simulink model "gm_hdl_model_fixed_vnl"  (R2024a)
settings: Solver=FixedStepDiscrete  StartTime=0.0  StopTime=SIM_TIME  RelTol=1e-3
undefined symbols (not defined in the file or in its folder): a, b, BUFFER_LEN, c, SAMPLING_FREQ, signal_1
libraries: hdlsllib x41, simulink x16, dspsigops x15, simulink_extras x5, dsphdlxfrm2 x2, dspsrcs4 x1
(part 2 of 3)

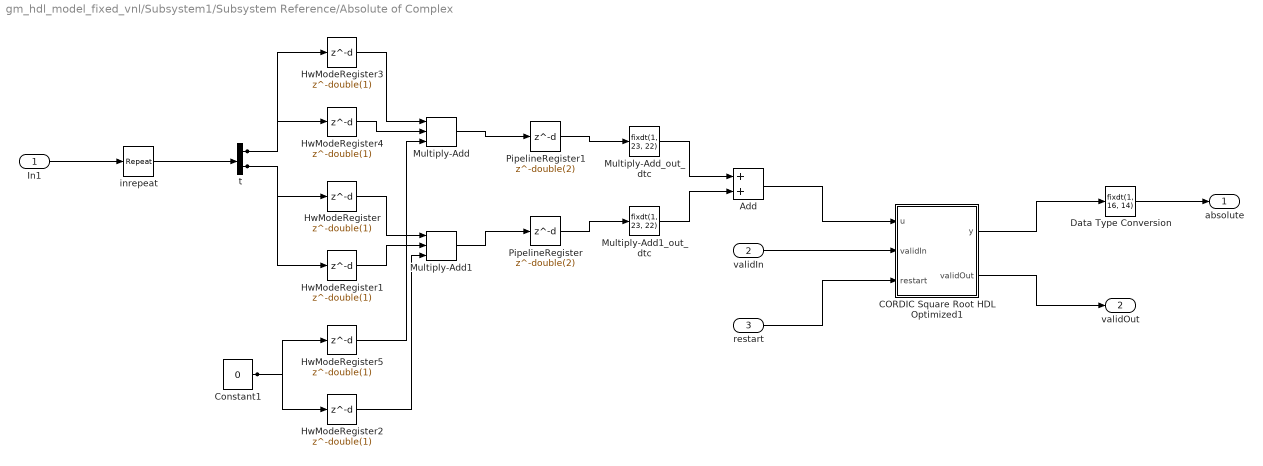
== system gm_hdl_model_fixed_vnl/Subsystem1/Subsystem Reference/Absolute of Complex ==
  In1 : Inport  OutDataTypeStr=fixdt(1, 12, 11)  PortDimensions=[2]  SampleTime=1e-08
  validIn : Inport  Port=2  OutDataTypeStr=boolean  PortDimensions=1  SampleTime=1e-08
  restart : Inport  Port=3  OutDataTypeStr=boolean  PortDimensions=1  SampleTime=1e-08
  Add : Sum  OutDataTypeStr=fixdt(1, 24, 22)  AccumDataTypeStr=fixdt(1, 24, 22)  SampleTime=5e-09
  CORDIC Square Root HDL Optimized1 : Subsystem  mask(CORDIC Square Root HDL Optimized){autoMaximumShiftVal=on, maximumShiftValue=double(10), nIterPerReg=double(1)}
      mask prompts: autoMaximumShiftVal "fixed:emblib:AutoCORDICMaxShiftValue"; maximumShiftValue "fixed:emblib:CORDICMaxShiftValue"; nIterPerReg "fixed:emblib:NumberOfIterationsPerReg"
      mask help: fixed:emblib:CORDICSquareRootHDLFullDescription
      mask Help: eval('embblk.embhelp(gcb)')
      mask Callback autoMaximumShiftVal:
      | autoMaxShiftVal = get_param(gcb,'autoMaximumShiftVal');
      | if strcmp(autoMaxShiftVal,'on')
      |     set_param(gcb,'MaskVisibilities',{'on','off','on'});
      | else
      |     set_param(gcb,'MaskVisibilities',{'on','on','on'});
      | end
      mask Display: disp('CORDIC Square Root\nHDL Optimized')
  Constant1 : Constant  Value=0  OutDataTypeStr=fixdt(1, 12, 11)  SampleTime=5e-09
  Data Type Conversion : DataTypeConversion  OutDataTypeStr=fixdt(1, 16, 14)  SampleTime=5e-09  SaturateOnIntegerOverflow=off  RndMeth=Floor
  HwModeRegister{,1..5} (6 alike) : Delay  DelayLength=double(1)  InitialCondition=0  SampleTime=5e-09
  Multiply-Add : hdlsllib/HDL Operations/Multiply-Add  Function=c+(a.*b)  datatype=fixdt(1, 25, 22)  DoSatur=off  FMA=off
  Multiply-Add1 : hdlsllib/HDL Operations/Multiply-Add  Function=c+(a.*b)  datatype=fixdt(1, 25, 22)  DoSatur=off  FMA=off
  Multiply-Add1_out_dtc : DataTypeConversion  OutDataTypeStr=fixdt(1, 23, 22)  SampleTime=5e-09  SaturateOnIntegerOverflow=off  RndMeth=Floor
  Multiply-Add_out_dtc : DataTypeConversion  OutDataTypeStr=fixdt(1, 23, 22)  SampleTime=5e-09  SaturateOnIntegerOverflow=off  RndMeth=Floor
  PipelineRegister : Delay  DelayLength=double(2)  InitialCondition=0  SampleTime=5e-09
  PipelineRegister1 : Delay  DelayLength=double(2)  InitialCondition=0  SampleTime=5e-09
  inrepeat : dspsigops/Repeat  FactorSource=Dialog parameter  N=double(2)  Nmax=16  RateOptions=Allow multirate processing  ic=0  mode=Unused parameter value
  t : Demux  Outputs=2
  absolute : Outport  SampleTime=5e-09
  validOut : Outport  Port=2  SampleTime=1e-08
  wires:
  HwModeRegister5/1 -> Multiply-Add/3
  HwModeRegister4/1 -> Multiply-Add/2
  HwModeRegister3/1 -> Multiply-Add/1
  Multiply-Add/1 -> PipelineRegister1/1
  HwModeRegister2/1 -> Multiply-Add1/3
  HwModeRegister1/1 -> Multiply-Add1/2
  HwModeRegister/1 -> Multiply-Add1/1
  Multiply-Add1/1 -> PipelineRegister/1
  PipelineRegister1/1 -> Multiply-Add_out_dtc/1
  PipelineRegister/1 -> Multiply-Add1_out_dtc/1
  t/2 -> HwModeRegister1/1, HwModeRegister/1
  t/1 -> HwModeRegister4/1, HwModeRegister3/1
  Multiply-Add_out_dtc/1 -> Add/1
  Multiply-Add1_out_dtc/1 -> Add/2
  Constant1/1 -> HwModeRegister5/1, HwModeRegister2/1
  inrepeat/1 -> t/1
  CORDIC Square Root HDL Optimized1/1(y) -> Data Type Conversion/1
  Add/1 -> CORDIC Square Root HDL Optimized1/1(u)
  Data Type Conversion/1 -> absolute/1
  CORDIC Square Root HDL Optimized1/2(validOut) -> validOut/1
  restart/1 -> CORDIC Square Root HDL Optimized1/3(restart)
  validIn/1 -> CORDIC Square Root HDL Optimized1/2(validIn)
  In1/1 -> inrepeat/1

== system gm_hdl_model_fixed_vnl/Subsystem1/Subsystem Reference/CORDIC Square Root HDL Optimized ==
  u : Inport  OutDataTypeStr=fixdt(1, 22, 20)  SampleTime=1e-08
  validIn : Inport  Port=2  OutDataTypeStr=boolean  SampleTime=1e-08
  restart : Inport  Port=3  OutDataTypeStr=boolean  SampleTime=1e-08
  Bit Shift Arithmetic : Subsystem
  Cast to Union of Types : Subsystem
  Data Type Conversion : DataTypeConversion  OutDataTypeStr=fixdt(1,22,20)
  Synchronous Subsystem : Subsystem
  y : Outport  SampleTime=1e-08
  validOut : Outport  Port=2  SampleTime=1e-08
  wires:
  Bit Shift Arithmetic/1(y) -> Data Type Conversion/1
  Cast to Union of Types/1(Cout) -> Bit Shift Arithmetic/1(u)
  Synchronous Subsystem/4(validOut) -> validOut/1
  Synchronous Subsystem/3(isZero) -> Bit Shift Arithmetic/3(isZero)
  Synchronous Subsystem/2(eOut) -> Bit Shift Arithmetic/2(e)
  Synchronous Subsystem/1(dataOut) -> Cast to Union of Types/2(Cin)
  Data Type Conversion/1 -> y/1
  restart/1 -> Synchronous Subsystem/3(restart)
  validIn/1 -> Synchronous Subsystem/2(validIn)
  u/1 -> Cast to Union of Types/1(Xref), Synchronous Subsystem/1(u)

== system gm_hdl_model_fixed_vnl/Subsystem1/Subsystem Reference/Real Divide HDL Optimized ==
  num : Inport  OutDataTypeStr=fixdt(1, 17, 14)  SampleTime=1e-08
  den : Inport  Port=2  OutDataTypeStr=fixdt(1, 17, 14)  SampleTime=5e-09
  validIn : Inport  Port=3  OutDataTypeStr=boolean  SampleTime=1e-08
  Delay1 : Delay  DelayLength=double(1)  InitialCondition=0  SampleTime=1e-08
  Delay17 : Delay  DelayLength=double(1)  InitialCondition=0  SampleTime=1e-08
  ForEach - Real Divide_instance1 : Subsystem
  Reshape to original size : Subsystem
  Verify divide sizes : Subsystem
  in1_repeat : dspsigops/Repeat  FactorSource=Dialog parameter  N=double(2)  Nmax=16  RateOptions=Allow multirate processing  ic=0  mode=Unused parameter value
  y = u(1) : Subsystem
  y : Outport  SampleTime=1e-08
  validOut : Outport  Port=2  SampleTime=1e-08
  wires:
  in1_repeat/1 -> Verify divide sizes/2(numerator)
  Verify divide sizes/2(num) -> ForEach - Real Divide_instance1/2(num)
  Verify divide sizes/1(den) -> ForEach - Real Divide_instance1/1(den)
  den/1 -> Verify divide sizes/1(denominator)
  Reshape to original size/1(z) -> Delay17/1
  y = u(1)/1(y) -> Delay1/1
  Delay17/1 -> y/1
  Delay1/1 -> validOut/1
  ForEach - Real Divide_instance1/2(validOut) -> y = u(1)/1(u)
  ForEach - Real Divide_instance1/1(y) -> Reshape to original size/1(y)
  validIn/1 -> ForEach - Real Divide_instance1/3(validIn)
  num/1 -> in1_repeat/1, Reshape to original size/2(u)

== system gm_hdl_model_fixed_vnl/Subsystem1/Subsystem Reference/Sample and Hold ==
  In : Inport  OutDataTypeStr=fixdt(1, 16, 14)
  Trigger : TriggerPort  VariantControl=(inherit)  OutDataTypeStr=boolean
  " " : Outport  InitialOutput=0
  wires:
  In/1 -> " "/1

== system gm_hdl_model_fixed_vnl/Subsystem1/Subsystem Reference/Sample and Hold1 ==
  In : Inport  OutDataTypeStr=fixdt(1, 18, 10)
  Trigger : TriggerPort  VariantControl=(inherit)  OutDataTypeStr=boolean
  " " : Outport  InitialOutput=0
  wires:
  In/1 -> " "/1

== system gm_hdl_model_fixed_vnl/Subsystem1/Subsystem Reference/Sample and Hold2 ==
  In : Inport  OutDataTypeStr=fixdt(1, 22, 20)
  Trigger : TriggerPort  VariantControl=(inherit)  OutDataTypeStr=boolean
  " " : Outport  InitialOutput=0
  wires:
  In/1 -> " "/1

== system gm_hdl_model_fixed_vnl/Subsystem1/Subsystem Reference/Select_Freq ==
  enb : Inport  OutDataTypeStr=boolean  PortDimensions=1  SampleTime=1e-08
  AND : Logic  AllPortsSameDT=off  OutDataTypeStr=boolean  SampleTime=1e-08
  Constant : Constant  Value=0  OutDataTypeStr=boolean  SampleTime=1e-08
  Constant1 : Constant  OutDataTypeStr=boolean  SampleTime=1e-08
  HDL Counter_controlled : Subsystem
  NOT : Logic  Operator=NOT  Inputs=1  AllPortsSameDT=off  OutDataTypeStr=boolean  SampleTime=1e-08
  Switch : Switch  Criteria=u2 > Threshold  Threshold=double(9)  OutDataTypeStr=boolean  SampleTime=1e-08  SaturateOnIntegerOverflow=off  InputSameDT=off
  Switch1 : Switch  Criteria=u2 > Threshold  Threshold=double(1024)  OutDataTypeStr=boolean  SampleTime=1e-08  SaturateOnIntegerOverflow=off  InputSameDT=off
  adder : Sum  OutDataTypeStr=fixdt(0, 12, 0)  AccumDataTypeStr=fixdt(0, 12, 0)  SampleTime=1e-08
  compare : simulink/Logic and Bit Operations/Compare To Constant  relop===  const="fi(0,0,12,0,\"hex\",\"800\")"  OutDataTypeStr=boolean
  const : Constant  Value=0  VectorParams1D=off  OutDataTypeStr=fixdt(0, 12, 0)  SampleTime=1e-08
  countFrom : Constant  Value=0  VectorParams1D=off  OutDataTypeStr=fixdt(0, 12, 0)  SampleTime=1e-08
  delayMatch : Delay  DelayLength=double(2)  InitialCondition=0  SampleTime=1e-08
  stateControl : Constant  OutDataTypeStr=boolean  SampleTime=1e-08
  step_value : Constant  VectorParams1D=off  OutDataTypeStr=fixdt(0, 12, 0)  SampleTime=1e-08
  switch : Switch  Criteria=u2 ~= 0  Threshold=double(0)  OutDataTypeStr=fixdt(0, 12, 0)  SampleTime=1e-08  SaturateOnIntegerOverflow=off  InputSameDT=off
  switchEnable : MultiPortSwitch  DataPortOrder=Zero-based contiguous  Inputs=2  DiagnosticForDefault=None  zeroidx=on  OutDataTypeStr=fixdt(0, 12, 0)  SampleTime=1e-08  SaturateOnIntegerOverflow=off  InputSameDT=off
  switchReset : Switch  Criteria=u2 ~= 0  Threshold=double(0)  OutDataTypeStr=fixdt(0, 12, 0)  SampleTime=1e-08  SaturateOnIntegerOverflow=off  InputSameDT=off
  Out1 : Outport  OutDataTypeStr=boolean  SampleTime=1e-08
  wires:
  switchEnable/1 -> switchReset/3
  switch/1 -> switchEnable/3
  compare/1 -> switch/2
  adder/1 -> switch/3
  switchReset/1 -> HDL Counter_controlled/1(in0)
  NOT/1 -> switchReset/2
  const/1 -> switchReset/1
  countFrom/1 -> switch/1
  step_value/1 -> adder/2
  delayMatch/1 -> HDL Counter_controlled/Enable
  HDL Counter_controlled/1(out0) -> Switch1/2, Switch/2, switchEnable/2, compare/1, adder/1
  stateControl/1 -> delayMatch/1
  Switch/1 -> AND/1
  Constant1/1 -> Switch1/3, Switch/1
  Switch1/1 -> AND/2
  Constant/1 -> Switch1/1, Switch/3
  AND/1 -> Out1/1
  enb/1 -> switchEnable/1, NOT/1

== system gm_hdl_model_fixed_vnl/Subsystem1/myRMS/CORDIC Square Root HDL Optimized ==
  u : Inport  OutDataTypeStr=fixdt(0, 16, 7)  SampleTime=1e-08
  validIn : Inport  Port=2  OutDataTypeStr=boolean  SampleTime=1e-08
  restart : Inport  Port=3  OutDataTypeStr=boolean  SampleTime=1e-08
  Bit Shift Arithmetic : Subsystem
  Cast to Union of Types : Subsystem
  Data Type Conversion : DataTypeConversion  OutDataTypeStr=fixdt(0, 16, 7)  RndMeth=Nearest  SampleTime=1e-08  SaturateOnIntegerOverflow=off
  Synchronous Subsystem : Subsystem
  y : Outport  SampleTime=1e-08
  validOut : Outport  Port=2  SampleTime=1e-08
  wires:
  Bit Shift Arithmetic/1(y) -> Data Type Conversion/1
  Cast to Union of Types/1(Cout) -> Bit Shift Arithmetic/1(u)
  Synchronous Subsystem/4(validOut) -> validOut/1
  Synchronous Subsystem/3(isZero) -> Bit Shift Arithmetic/3(isZero)
  Synchronous Subsystem/2(eOut) -> Bit Shift Arithmetic/2(e)
  Synchronous Subsystem/1(dataOut) -> Cast to Union of Types/2(Cin)
  Data Type Conversion/1 -> y/1
  restart/1 -> Synchronous Subsystem/3(restart)
  validIn/1 -> Synchronous Subsystem/2(validIn)
  u/1 -> Cast to Union of Types/1(Xref), Synchronous Subsystem/1(u)

== system gm_hdl_model_fixed_vnl/Subsystem1/myRMS/Sample and Hold ==
  In : Inport  OutDataTypeStr=fixdt(0, 16, 7)
  Trigger : TriggerPort  VariantControl=(inherit)  OutDataTypeStr=boolean
  " " : Outport  InitialOutput=0
  wires:
  In/1 -> " "/1

== system gm_hdl_model_fixed_vnl/Subsystem1/Subsystem Reference/Absolute of Complex/CORDIC Square Root HDL Optimized1 ==
  u : Inport  OutDataTypeStr=fixdt(1, 24, 22)  SampleTime=5e-09
  validIn : Inport  Port=2  OutDataTypeStr=boolean  SampleTime=1e-08
  restart : Inport  Port=3  OutDataTypeStr=boolean  SampleTime=1e-08
  Bit Shift Arithmetic : Subsystem
  Cast to Union of Types : Subsystem
  Data Type Conversion : DataTypeConversion  OutDataTypeStr=fixdt(1,24,22)
  Synchronous Subsystem : Subsystem
  delayMatch : Delay  DelayLength=double(4)  InitialCondition=0  SampleTime=5e-09
  in1_repeat : dspsigops/Repeat  FactorSource=Dialog parameter  N=double(2)  Nmax=16  RateOptions=Allow multirate processing  ic=0  mode=Unused parameter value
  in2_repeat : dspsigops/Repeat  FactorSource=Dialog parameter  N=double(2)  Nmax=16  RateOptions=Allow multirate processing  ic=0  mode=Unused parameter value
  in3_repeat : dspsigops/Repeat  FactorSource=Dialog parameter  N=double(2)  Nmax=16  RateOptions=Allow multirate processing  ic=0  mode=Unused parameter value
  y : Outport  SampleTime=5e-09
  validOut : Outport  Port=2  SampleTime=1e-08
  wires:
  Bit Shift Arithmetic/1(y) -> Data Type Conversion/1
  Cast to Union of Types/1(Cout) -> Bit Shift Arithmetic/1(u)
  u/1 -> Synchronous Subsystem/1(u), delayMatch/1
  in3_repeat/1 -> Bit Shift Arithmetic/3(isZero)
  in2_repeat/1 -> Bit Shift Arithmetic/2(e)
  in1_repeat/1 -> Cast to Union of Types/2(Cin)
  Data Type Conversion/1 -> y/1
  delayMatch/1 -> Cast to Union of Types/1(Xref)
  Synchronous Subsystem/4(validOut) -> validOut/1
  Synchronous Subsystem/3(isZero) -> in3_repeat/1
  Synchronous Subsystem/2(eOut) -> in2_repeat/1
  Synchronous Subsystem/1(dataOut) -> in1_repeat/1
  restart/1 -> Synchronous Subsystem/3(restart)
  validIn/1 -> Synchronous Subsystem/2(validIn)

== system gm_hdl_model_fixed_vnl/Subsystem1/Subsystem Reference/CORDIC Square Root HDL Optimized/Bit Shift Arithmetic ==
  u : Inport  OutDataTypeStr=fixdt(1, 22, 20)  PortDimensions=1  SampleTime=1e-08
  e : Inport  Port=2  OutDataTypeStr=int32  PortDimensions=1  SampleTime=1e-08
  isZero : Inport  Port=3  OutDataTypeStr=boolean  PortDimensions=1  SampleTime=1e-08
  embmathops_c6_sxviEMGenxpVSWTChSq0GHG_Bit_Shift_Arithmetic : MATLAB Function  TreatAsAtomicUnit=on
      settings: LibrarySourceBlock=embmathops/CORDIC Square Root HDL Optimized/Bit Shift Arithmetic
  y : Outport  SampleTime=1e-08  VectorParamsAs1DForOutWhenUnconnected=off
  wires:
  embmathops_c6_sxviEMGenxpVSWTChSq0GHG_Bit_Shift_Arithmetic/1(y) -> y/1
  isZero/1 -> embmathops_c6_sxviEMGenxpVSWTChSq0GHG_Bit_Shift_Arithmetic/3(isZero)
  e/1 -> embmathops_c6_sxviEMGenxpVSWTChSq0GHG_Bit_Shift_Arithmetic/2(e)
  u/1 -> embmathops_c6_sxviEMGenxpVSWTChSq0GHG_Bit_Shift_Arithmetic/1(u)

== system gm_hdl_model_fixed_vnl/Subsystem1/Subsystem Reference/CORDIC Square Root HDL Optimized/Cast to Union of Types ==
  Xref : Inport  OutDataTypeStr=fixdt(1, 22, 20)  SampleTime=1e-08
  Cin : Inport  Port=2  OutDataTypeStr=fixdt(1, 22, 20)  SampleTime=1e-08
  slutils_c1_sUkuwzpcxqKl25e4GzDa0OH_Cast_to_Union_of_Types : MATLAB Function
      settings: LibrarySourceBlock=slutils/Cast to Union of Types
  Cout : Outport  SampleTime=1e-08
  wires:
  slutils_c1_sUkuwzpcxqKl25e4GzDa0OH_Cast_to_Union_of_Types/1(Cout) -> Cout/1
  Cin/1 -> slutils_c1_sUkuwzpcxqKl25e4GzDa0OH_Cast_to_Union_of_Types/2(Cin)
  Xref/1 -> slutils_c1_sUkuwzpcxqKl25e4GzDa0OH_Cast_to_Union_of_Types/1(Xref)

== system gm_hdl_model_fixed_vnl/Subsystem1/Subsystem Reference/CORDIC Square Root HDL Optimized/Synchronous Subsystem ==
  u : Inport  OutDataTypeStr=fixdt(1, 22, 20)  PortDimensions=1  SampleTime=1e-08
  validIn : Inport  Port=2  OutDataTypeStr=boolean  PortDimensions=1  SampleTime=1e-08
  restart : Inport  Port=3  OutDataTypeStr=boolean  PortDimensions=1  SampleTime=1e-08
  StateControl : StateControl  StateControl=Synchronous
  cordicSquareRootHDL : Subsystem
  dataOut : Outport  SampleTime=1e-08  VectorParamsAs1DForOutWhenUnconnected=off
  eOut : Outport  Port=2  SampleTime=1e-08  VectorParamsAs1DForOutWhenUnconnected=off
  isZero : Outport  Port=3  SampleTime=1e-08  VectorParamsAs1DForOutWhenUnconnected=off
  validOut : Outport  Port=4  SampleTime=1e-08  VectorParamsAs1DForOutWhenUnconnected=off
  wires:
  cordicSquareRootHDL/4(validOut) -> validOut/1
  cordicSquareRootHDL/3(isZero) -> isZero/1
  cordicSquareRootHDL/2(eOut) -> eOut/1
  cordicSquareRootHDL/1(dataOut) -> dataOut/1
  restart/1 -> cordicSquareRootHDL/3(restart)
  validIn/1 -> cordicSquareRootHDL/2(validIn)
  u/1 -> cordicSquareRootHDL/1(u)

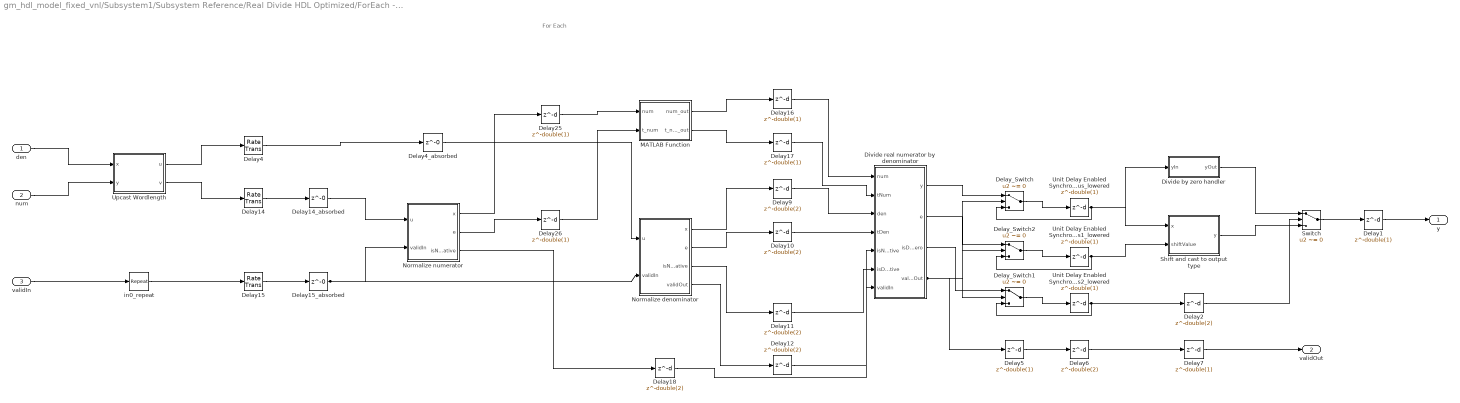
== system gm_hdl_model_fixed_vnl/Subsystem1/Subsystem Reference/Real Divide HDL Optimized/ForEach - Real Divide_instance1 ==
  note: For Each
  den : Inport  OutDataTypeStr=fixdt(1, 17, 14)  PortDimensions=1  SampleTime=5e-09
  num : Inport  Port=2  OutDataTypeStr=fixdt(1, 17, 14)  PortDimensions=1  SampleTime=5e-09
  validIn : Inport  Port=3  OutDataTypeStr=boolean  PortDimensions=1  SampleTime=1e-08
  Delay{1,5,7,16..17,25..26} (7 alike) : Delay  DelayLength=double(1)  InitialCondition=0  SampleTime=1e-08
  Delay{2,6,9..12,18} (7 alike) : Delay  DelayLength=double(2)  InitialCondition=0  SampleTime=1e-08
  Delay14 : RateTransition  OutPortSampleTimeOpt=Multiple of input port sample time  OutPortSampleTimeMultiple=2
  Delay14_absorbed : Delay  DelayLength=0
  Delay15 : RateTransition  OutPortSampleTimeOpt=Multiple of input port sample time  OutPortSampleTimeMultiple=2
  Delay15_absorbed : Delay  DelayLength=0
  Delay4 : RateTransition  OutPortSampleTimeOpt=Multiple of input port sample time  OutPortSampleTimeMultiple=2
  Delay4_absorbed : Delay  DelayLength=0
  Delay_Switch : Switch  Criteria=u2 ~= 0  Threshold=double(0)  OutDataTypeStr=fixdt(1, 17, 15)  SampleTime=1e-08  SaturateOnIntegerOverflow=off  InputSameDT=off
  Delay_Switch1 : Switch  Criteria=u2 ~= 0  Threshold=double(0)  OutDataTypeStr=boolean  SampleTime=1e-08  SaturateOnIntegerOverflow=off  InputSameDT=off
  Delay_Switch2 : Switch  Criteria=u2 ~= 0  Threshold=double(0)  OutDataTypeStr=fixdt(1, 34, 0)  SampleTime=1e-08  SaturateOnIntegerOverflow=off  InputSameDT=off
  Divide by zero handler : Subsystem
  Divide real numerator by denominator : Subsystem
  MATLAB Function : Subsystem
  Normalize denominator : Subsystem  mask(Real Normalizer HDL Optimized){}
      mask help: fixed:emblib:RealNormalizerFullDescription
      mask Help: For internal use only. This feature is intentionally undocumented. Its behavior may change, or it may be removed in a future release.
      mask Display:
      | text(0.5,0.8,'u ~= 0','texmode','on','HorizontalAlignment','center')
      | text(0.5,0.6,'x = 2^e |u|','texmode','on','HorizontalAlignment','center')
      | text(0.5,0.4,'1 \leq x < 2','texmode','on','HorizontalAlignment','center')
      | text(0.5,0.2,'isNegative = u<0','texmode','on','HorizontalAlignment','center')
  Normalize numerator : Subsystem  mask(Real Normalizer HDL Optimized){}
      mask help: fixed:emblib:RealNormalizerFullDescription
      mask Help: For internal use only. This feature is intentionally undocumented. Its behavior may change, or it may be removed in a future release.
      mask Display:
      | text(0.5,0.8,'u ~= 0','texmode','on','HorizontalAlignment','center')
      | text(0.5,0.6,'x = 2^e |u|','texmode','on','HorizontalAlignment','center')
      | text(0.5,0.4,'1 \leq x < 2','texmode','on','HorizontalAlignment','center')
      | text(0.5,0.2,'isNegative = u<0','texmode','on','HorizontalAlignment','center')
  Shift and cast to output type : Subsystem  mask{OutputType=OutputType}
      mask prompts: OutputType "fixed:emblib:OutputPrototype"
  Switch : Switch  Criteria=u2 ~= 0  Threshold=double(0)  OutDataTypeStr=fixdt(1, 18, 10)  SampleTime=1e-08  SaturateOnIntegerOverflow=off  InputSameDT=off
  Unit Delay Enabled Synchronous1_lowered : Delay  DelayLength=double(1)  InitialCondition=0  SampleTime=1e-08
  Unit Delay Enabled Synchronous2_lowered : Delay  DelayLength=double(1)  InitialCondition=0  SampleTime=1e-08
  Unit Delay Enabled Synchronous_lowered : Delay  DelayLength=double(1)  InitialCondition=0  SampleTime=1e-08
  Upcast Wordlength : Subsystem
  in0_repeat : dspsigops/Repeat  FactorSource=Dialog parameter  N=double(2)  Nmax=16  RateOptions=Allow multirate processing  ic=0  mode=Unused parameter value
  y : Outport  SampleTime=1e-08
  validOut : Outport  Port=2  SampleTime=1e-08
  wires:
  Delay15/1 -> Delay15_absorbed/1
  Delay_Switch1/1 -> Unit Delay Enabled Synchronous2_lowered/1
  Unit Delay Enabled Synchronous2_lowered/1 -> Delay2/1, Delay_Switch1/3
  Delay_Switch/1 -> Unit Delay Enabled Synchronous_lowered/1
  Unit Delay Enabled Synchronous_lowered/1 -> Shift and cast to output type/1(x), Divide by zero handler/1(yIn), Delay_Switch/3
  Delay_Switch2/1 -> Unit Delay Enabled Synchronous1_lowered/1
  Unit Delay Enabled Synchronous1_lowered/1 -> Shift and cast to output type/2(shiftValue), Delay_Switch2/3
  Delay14_absorbed/1 -> Normalize numerator/1(u)
  Delay4_absorbed/1 -> Normalize denominator/1(u)
  Delay14/1 -> Delay14_absorbed/1
  Delay4/1 -> Delay4_absorbed/1
  Upcast Wordlength/2(v) -> Delay14/1
  Upcast Wordlength/1(u) -> Delay4/1
  in0_repeat/1 -> Delay15/1
  Delay15_absorbed/1 -> Normalize numerator/2(validIn), Normalize denominator/2(validIn)
  num/1 -> Upcast Wordlength/2(y)
  den/1 -> Upcast Wordlength/1(x)
  MATLAB Function/2(t_num_out) -> Delay17/1
  MATLAB Function/1(num_out) -> Delay16/1
  Switch/1 -> Delay1/1
  Delay26/1 -> MATLAB Function/2(t_num)
  Delay25/1 -> MATLAB Function/1(num)
  Delay5/1 -> Delay6/1
  Delay2/1 -> Switch/2
  Delay6/1 -> Delay7/1
  Delay17/1 -> Divide real numerator by denominator/2(tNum)
  Delay16/1 -> Divide real numerator by denominator/1(num)
  Delay10/1 -> Divide real numerator by denominator/4(tDen)
  Delay11/1 -> Divide real numerator by denominator/6(isDenNegative)
  Delay12/1 -> Divide real numerator by denominator/7(validIn)
  Delay18/1 -> Divide real numerator by denominator/5(isNumNegative)
  Delay9/1 -> Divide real numerator by denominator/3(den)
  Delay1/1 -> y/1
  Delay7/1 -> validOut/1
  Divide by zero handler/1(yOut) -> Switch/1
  Divide real numerator by denominator/4(validOut) -> Delay_Switch2/2, Delay_Switch1/2, Delay_Switch/2, Delay5/1
  Divide real numerator by denominator/3(isDenZero) -> Delay_Switch1/1
  Divide real numerator by denominator/2(e) -> Delay_Switch2/1
  Divide real numerator by denominator/1(y) -> Delay_Switch/1
  Normalize denominator/4(validOut) -> Delay12/1
  Normalize denominator/3(isNegative) -> Delay11/1
  Normalize denominator/2(e) -> Delay10/1
  Normalize denominator/1(x) -> Delay9/1
  Normalize numerator/3(isNegative) -> Delay18/1
  Normalize numerator/2(e) -> Delay26/1
  Normalize numerator/1(x) -> Delay25/1
  Shift and cast to output type/1(y) -> Switch/3
  validIn/1 -> in0_repeat/1

== system gm_hdl_model_fixed_vnl/Subsystem1/Subsystem Reference/Real Divide HDL Optimized/Reshape to original size ==
  y : Inport  OutDataTypeStr=fixdt(1, 18, 10)  PortDimensions=1  SampleTime=1e-08
  u : Inport  Port=2  OutDataTypeStr=fixdt(1, 17, 14)  PortDimensions=1  SampleTime=1e-08
  delayMatch : Delay  DelayLength=double(1)  InitialCondition=0  SampleTime=1e-08
  embreciprocals_c11_Reshape_to_original_size : MATLAB Function  TreatAsAtomicUnit=on
      settings: LibrarySourceBlock=embreciprocals/Real Divide HDL Optimized/Reshape to original size
  z : Outport  SampleTime=1e-08
  wires:
  u/1 -> delayMatch/1
  embreciprocals_c11_Reshape_to_original_size/1(z) -> z/1
  delayMatch/1 -> embreciprocals_c11_Reshape_to_original_size/2(u)
  y/1 -> embreciprocals_c11_Reshape_to_original_size/1(y)

== system gm_hdl_model_fixed_vnl/Subsystem1/Subsystem Reference/Real Divide HDL Optimized/Verify divide sizes ==
  denominator : Inport  OutDataTypeStr=fixdt(1, 17, 14)  PortDimensions=1  SampleTime=5e-09
  numerator : Inport  Port=2  OutDataTypeStr=fixdt(1, 17, 14)  PortDimensions=1  SampleTime=5e-09
  delayMatch : Delay  DelayLength=double(3)  InitialCondition=0  SampleTime=5e-09
  embreciprocals_c19_Verify_divide_sizes : MATLAB Function  TreatAsAtomicUnit=on
      settings: LibrarySourceBlock=embreciprocals/Real Divide HDL Optimized/Verify divide sizes
  den : Outport  SampleTime=5e-09
  num : Outport  Port=2  SampleTime=5e-09
  wires:
  numerator/1 -> delayMatch/1
  embreciprocals_c19_Verify_divide_sizes/2(num) -> num/1
  embreciprocals_c19_Verify_divide_sizes/1(den) -> den/1
  delayMatch/1 -> embreciprocals_c19_Verify_divide_sizes/2(numerator)
  denominator/1 -> embreciprocals_c19_Verify_divide_sizes/1(denominator)

== system gm_hdl_model_fixed_vnl/Subsystem1/Subsystem Reference/Real Divide HDL Optimized/y = u(1) ==
  u : Inport  OutDataTypeStr=boolean  PortDimensions=1  SampleTime=1e-08
  embreciprocals_c16_y___u_1_ : MATLAB Function  TreatAsAtomicUnit=on
      settings: LibrarySourceBlock=embreciprocals/Real Divide HDL Optimized/y = u(1)
  y : Outport  SampleTime=1e-08
  wires:
  embreciprocals_c16_y___u_1_/1(y) -> y/1
  u/1 -> embreciprocals_c16_y___u_1_/1(u)

== system gm_hdl_model_fixed_vnl/Subsystem1/Subsystem Reference/Select_Freq/HDL Counter_controlled ==
  in0 : Inport  OutDataTypeStr=fixdt(0, 12, 0)  SampleTime=1e-08
  stateControl : EnablePort  OutDataTypeStr=boolean
  HDL Counter : Delay  DelayLength=double(1)  InitialCondition=0  SampleTime=1e-08
  out0 : Outport  OutDataTypeStr=fixdt(0, 12, 0)  SampleTime=1e-08
  wires:
  in0/1 -> HDL Counter/1
  HDL Counter/1 -> out0/1

== system gm_hdl_model_fixed_vnl/Subsystem1/myRMS/CORDIC Square Root HDL Optimized/Bit Shift Arithmetic ==
  u : Inport  OutDataTypeStr=fixdt(1, 24, 14)  PortDimensions=1  SampleTime=1e-08
  e : Inport  Port=2  OutDataTypeStr=int32  PortDimensions=1  SampleTime=1e-08
  isZero : Inport  Port=3  OutDataTypeStr=boolean  PortDimensions=1  SampleTime=1e-08
  embmathops_c6_st99WwhDyWfnOmuPiiKPkxE_Bit_Shift_Arithmetic : MATLAB Function  TreatAsAtomicUnit=on
      settings: LibrarySourceBlock=embmathops/CORDIC Square Root HDL Optimized/Bit Shift Arithmetic
  y : Outport  SampleTime=1e-08  VectorParamsAs1DForOutWhenUnconnected=off
  wires:
  embmathops_c6_st99WwhDyWfnOmuPiiKPkxE_Bit_Shift_Arithmetic/1(y) -> y/1
  isZero/1 -> embmathops_c6_st99WwhDyWfnOmuPiiKPkxE_Bit_Shift_Arithmetic/3(isZero)
  e/1 -> embmathops_c6_st99WwhDyWfnOmuPiiKPkxE_Bit_Shift_Arithmetic/2(e)
  u/1 -> embmathops_c6_st99WwhDyWfnOmuPiiKPkxE_Bit_Shift_Arithmetic/1(u)

== system gm_hdl_model_fixed_vnl/Subsystem1/myRMS/CORDIC Square Root HDL Optimized/Cast to Union of Types ==
  Xref : Inport  OutDataTypeStr=fixdt(0, 16, 7)  SampleTime=1e-08
  Cin : Inport  Port=2  OutDataTypeStr=fixdt(1, 16, 14)  SampleTime=1e-08
  slutils_c1_sjX4rJHbVvOr6YSpugZXv9B_Cast_to_Union_of_Types : MATLAB Function
      settings: LibrarySourceBlock=slutils/Cast to Union of Types
  Cout : Outport  SampleTime=1e-08
  wires:
  slutils_c1_sjX4rJHbVvOr6YSpugZXv9B_Cast_to_Union_of_Types/1(Cout) -> Cout/1
  Cin/1 -> slutils_c1_sjX4rJHbVvOr6YSpugZXv9B_Cast_to_Union_of_Types/2(Cin)
  Xref/1 -> slutils_c1_sjX4rJHbVvOr6YSpugZXv9B_Cast_to_Union_of_Types/1(Xref)

== system gm_hdl_model_fixed_vnl/Subsystem1/myRMS/CORDIC Square Root HDL Optimized/Synchronous Subsystem ==
  u : Inport  OutDataTypeStr=fixdt(0, 16, 7)  PortDimensions=1  SampleTime=1e-08
  validIn : Inport  Port=2  OutDataTypeStr=boolean  PortDimensions=1  SampleTime=1e-08
  restart : Inport  Port=3  OutDataTypeStr=boolean  PortDimensions=1  SampleTime=1e-08
  StateControl : StateControl  StateControl=Synchronous
  cordicSquareRootHDL : Subsystem
  dataOut : Outport  SampleTime=1e-08  VectorParamsAs1DForOutWhenUnconnected=off
  eOut : Outport  Port=2  SampleTime=1e-08  VectorParamsAs1DForOutWhenUnconnected=off
  isZero : Outport  Port=3  SampleTime=1e-08  VectorParamsAs1DForOutWhenUnconnected=off
  validOut : Outport  Port=4  SampleTime=1e-08  VectorParamsAs1DForOutWhenUnconnected=off
  wires:
  cordicSquareRootHDL/4(validOut) -> validOut/1
  cordicSquareRootHDL/3(isZero) -> isZero/1
  cordicSquareRootHDL/2(eOut) -> eOut/1
  cordicSquareRootHDL/1(dataOut) -> dataOut/1
  restart/1 -> cordicSquareRootHDL/3(restart)
  validIn/1 -> cordicSquareRootHDL/2(validIn)
  u/1 -> cordicSquareRootHDL/1(u)

== system gm_hdl_model_fixed_vnl/Subsystem1/Subsystem Reference/Absolute of Complex/CORDIC Square Root HDL Optimized1/Bit Shift Arithmetic ==
  u : Inport  OutDataTypeStr=fixdt(1, 24, 22)  PortDimensions=1  SampleTime=5e-09
  e : Inport  Port=2  OutDataTypeStr=int32  PortDimensions=1  SampleTime=5e-09
  isZero : Inport  Port=3  OutDataTypeStr=boolean  PortDimensions=1  SampleTime=5e-09
  delayMatch : Delay  DelayLength=double(3)  InitialCondition=0  SampleTime=5e-09
  delayMatch1 : Delay  DelayLength=double(3)  InitialCondition=0  SampleTime=5e-09
  embmathops_c6_s5qJlWhB5AyunXvC1Wsa7cH_Bit_Shift_Arithmetic : MATLAB Function  TreatAsAtomicUnit=on
      settings: LibrarySourceBlock=embmathops/CORDIC Square Root HDL Optimized/Bit Shift Arithmetic
  y : Outport  SampleTime=5e-09  VectorParamsAs1DForOutWhenUnconnected=off
  wires:
  isZero/1 -> delayMatch1/1
  e/1 -> delayMatch/1
  embmathops_c6_s5qJlWhB5AyunXvC1Wsa7cH_Bit_Shift_Arithmetic/1(y) -> y/1
  delayMatch1/1 -> embmathops_c6_s5qJlWhB5AyunXvC1Wsa7cH_Bit_Shift_Arithmetic/3(isZero)
  delayMatch/1 -> embmathops_c6_s5qJlWhB5AyunXvC1Wsa7cH_Bit_Shift_Arithmetic/2(e)
  u/1 -> embmathops_c6_s5qJlWhB5AyunXvC1Wsa7cH_Bit_Shift_Arithmetic/1(u)

== system gm_hdl_model_fixed_vnl/Subsystem1/Subsystem Reference/Absolute of Complex/CORDIC Square Root HDL Optimized1/Cast to Union of Types ==
  Xref : Inport  OutDataTypeStr=fixdt(1, 24, 22)  SampleTime=5e-09
  Cin : Inport  Port=2  OutDataTypeStr=fixdt(1, 24, 22)  SampleTime=5e-09
  delayMatch : Delay  DelayLength=double(3)  InitialCondition=0  SampleTime=5e-09
  slutils_c1_sJq36p6JfwxqYYDPRgb8M6G_Cast_to_Union_of_Types : MATLAB Function
      settings: LibrarySourceBlock=slutils/Cast to Union of Types
  Cout : Outport  SampleTime=5e-09
  wires:
  Cin/1 -> delayMatch/1
  slutils_c1_sJq36p6JfwxqYYDPRgb8M6G_Cast_to_Union_of_Types/1(Cout) -> Cout/1
  delayMatch/1 -> slutils_c1_sJq36p6JfwxqYYDPRgb8M6G_Cast_to_Union_of_Types/2(Cin)
  Xref/1 -> slutils_c1_sJq36p6JfwxqYYDPRgb8M6G_Cast_to_Union_of_Types/1(Xref)

== system gm_hdl_model_fixed_vnl/Subsystem1/Subsystem Reference/Absolute of Complex/CORDIC Square Root HDL Optimized1/Synchronous Subsystem ==
  u : Inport  OutDataTypeStr=fixdt(1, 24, 22)  PortDimensions=1  SampleTime=5e-09
  validIn : Inport  Port=2  OutDataTypeStr=boolean  PortDimensions=1  SampleTime=1e-08
  restart : Inport  Port=3  OutDataTypeStr=boolean  PortDimensions=1  SampleTime=1e-08
  StateControl : StateControl  StateControl=Synchronous
  cordicSquareRootHDL : Subsystem
  dataOut : Outport  SampleTime=1e-08  VectorParamsAs1DForOutWhenUnconnected=off
  eOut : Outport  Port=2  SampleTime=1e-08  VectorParamsAs1DForOutWhenUnconnected=off
  isZero : Outport  Port=3  SampleTime=1e-08  VectorParamsAs1DForOutWhenUnconnected=off
  validOut : Outport  Port=4  SampleTime=1e-08  VectorParamsAs1DForOutWhenUnconnected=off
  wires:
  u/1 -> cordicSquareRootHDL/1(u)
  cordicSquareRootHDL/4(validOut) -> validOut/1
  cordicSquareRootHDL/3(isZero) -> isZero/1
  cordicSquareRootHDL/2(eOut) -> eOut/1
  cordicSquareRootHDL/1(dataOut) -> dataOut/1
  restart/1 -> cordicSquareRootHDL/3(restart)
  validIn/1 -> cordicSquareRootHDL/2(validIn)

== system gm_hdl_model_fixed_vnl/Subsystem1/Subsystem Reference/CORDIC Square Root HDL Optimized/Synchronous Subsystem/cordicSquareRootHDL ==
  u : Inport  OutDataTypeStr=fixdt(1, 22, 20)  PortDimensions=1  SampleTime=1e-08
  validIn : Inport  Port=2  OutDataTypeStr=boolean  PortDimensions=1  SampleTime=1e-08
  restart : Inport  Port=3  OutDataTypeStr=boolean  PortDimensions=1  SampleTime=1e-08
  delayMatch : Delay  DelayLength=double(4)  InitialCondition=0  SampleTime=1e-08
  delayMatch1 : Delay  DelayLength=double(4)  InitialCondition=0  SampleTime=1e-08
  embmathops_c2_skVmLPFzLIK224pVNfQB1qF_cordicSquareRootHDL_controlled : Subsystem
  stateControl : Constant  OutDataTypeStr=boolean  SampleTime=1e-08
  dataOut : Outport  SampleTime=1e-08  VectorParamsAs1DForOutWhenUnconnected=off
  eOut : Outport  Port=2  SampleTime=1e-08
  isZero : Outport  Port=3  SampleTime=1e-08
  validOut : Outport  Port=4  SampleTime=1e-08
  wires:
  stateControl/1 -> delayMatch1/1
  restart/1 -> delayMatch/1
  delayMatch1/1 -> embmathops_c2_skVmLPFzLIK224pVNfQB1qF_cordicSquareRootHDL_controlled/Enable
  embmathops_c2_skVmLPFzLIK224pVNfQB1qF_cordicSquareRootHDL_controlled/4(out3) -> validOut/1
  embmathops_c2_skVmLPFzLIK224pVNfQB1qF_cordicSquareRootHDL_controlled/3(out2) -> isZero/1
  embmathops_c2_skVmLPFzLIK224pVNfQB1qF_cordicSquareRootHDL_controlled/2(out1) -> eOut/1
  embmathops_c2_skVmLPFzLIK224pVNfQB1qF_cordicSquareRootHDL_controlled/1(out0) -> dataOut/1
  delayMatch/1 -> embmathops_c2_skVmLPFzLIK224pVNfQB1qF_cordicSquareRootHDL_controlled/3(in2)
  validIn/1 -> embmathops_c2_skVmLPFzLIK224pVNfQB1qF_cordicSquareRootHDL_controlled/2(in1)
  u/1 -> embmathops_c2_skVmLPFzLIK224pVNfQB1qF_cordicSquareRootHDL_controlled/1(in0)

== system gm_hdl_model_fixed_vnl/Subsystem1/Subsystem Reference/Real Divide HDL Optimized/ForEach - Real Divide_instance1/Divide by zero handler ==
  yIn : Inport  OutDataTypeStr=fixdt(1, 17, 15)  SampleTime=1e-08
  Compare To Zero : Subsystem  mask(Compare To Zero){relop=>=, OutDataTypeStr=boolean, ZeroCross=on}
      mask prompts: relop "Simulink:masks:Operator_MP"; OutDataTypeStr "Simulink:masks:OutputDataType_MP"; ZeroCross "Simulink:masks:EnableZerocrossingDetection_MP"
      mask help: Simulink:masks:CompareToZero_MD
      mask init:
      | OutDataTypeStr = 'boolean';
      | ZeroCross = 'on';
      | blkName = 'hdl_model_fixed/Subsystem1/Subsystem Reference/Real Divide HDL Optimized/ForEach - Real Divide/Divide by zero handler/Compare\nTo Zero';
      | relop = '>=';
      | setValue = 'boolean';
      mask TypeOptions relop: == | ~= | < | <= | >= | >
      mask TypeOptions OutDataTypeStr: Simulink:masks:uint8 | Simulink:masks:boolean
      mask Callback ZeroCross: sl('zeroCrossEnable', gcbh);
      mask Display: disp([relop,' 0'])
  Constant3 : Constant  Value=-128  OutDataTypeStr=fixdt(1, 18, 10)  SampleTime=1e-08
  Constant4 : Constant  Value=127.9990234375  OutDataTypeStr=fixdt(1, 18, 10)  SampleTime=1e-08
  Delay13 : Delay  DelayLength=double(1)  InitialCondition=0  SampleTime=1e-08
  Delay3 : Delay  DelayLength=double(1)  InitialCondition=0  SampleTime=1e-08
  Switch : Switch  Criteria=u2 > Threshold  Threshold=double(0)  OutDataTypeStr=fixdt(1, 18, 10)  SampleTime=1e-08  SaturateOnIntegerOverflow=off  InputSameDT=off
  yOut : Outport  SampleTime=1e-08
  wires:
  Compare To Zero/1(y) -> Delay13/1
  Switch/1 -> Delay3/1
  Constant3/1 -> Switch/3
  Constant4/1 -> Switch/1
  Delay13/1 -> Switch/2
  Delay3/1 -> yOut/1
  yIn/1 -> Compare To Zero/1(u)

== system gm_hdl_model_fixed_vnl/Subsystem1/Subsystem Reference/Real Divide HDL Optimized/ForEach - Real Divide_instance1/Divide real numerator by denominator ==
  num : Inport  OutDataTypeStr=fixdt(1, 17, 15)  SampleTime=1e-08
  tNum : Inport  Port=2  OutDataTypeStr=fixdt(1, 33, 0)  SampleTime=1e-08
  den : Inport  Port=3  OutDataTypeStr=fixdt(1, 17, 15)  SampleTime=1e-08
  tDen : Inport  Port=4  OutDataTypeStr=int32  SampleTime=1e-08
  isNumNegative : Inport  Port=5  OutDataTypeStr=boolean  SampleTime=1e-08
  isDenNegative : Inport  Port=6  OutDataTypeStr=boolean  SampleTime=1e-08
  validIn : Inport  Port=7  OutDataTypeStr=boolean  SampleTime=1e-08
  normalizedCORDICDivide : Subsystem
  y : Outport  SampleTime=1e-08
  e : Outport  Port=2  SampleTime=1e-08
  isDenZero : Outport  Port=3  SampleTime=1e-08
  validOut : Outport  Port=4  SampleTime=1e-08
  wires:
  validIn/1 -> normalizedCORDICDivide/7(validIn)
  isDenNegative/1 -> normalizedCORDICDivide/6(isDenNegative)
  isNumNegative/1 -> normalizedCORDICDivide/5(isNumNegative)
  tDen/1 -> normalizedCORDICDivide/4(tDen)
  den/1 -> normalizedCORDICDivide/2(den)
  tNum/1 -> normalizedCORDICDivide/3(tNum)
  num/1 -> normalizedCORDICDivide/1(num)
  normalizedCORDICDivide/4(validOut) -> validOut/1
  normalizedCORDICDivide/3(isDenZeroOut) -> isDenZero/1
  normalizedCORDICDivide/2(t) -> e/1
  normalizedCORDICDivide/1(y) -> y/1

== system gm_hdl_model_fixed_vnl/Subsystem1/Subsystem Reference/Real Divide HDL Optimized/ForEach - Real Divide_instance1/MATLAB Function ==
  num : Inport  OutDataTypeStr=fixdt(1, 17, 15)  PortDimensions=1  SampleTime=1e-08
  t_num : Inport  Port=2  OutDataTypeStr=int32  PortDimensions=1  SampleTime=1e-08
  embreciprocals_c13_MATLAB_Function : MATLAB Function  TreatAsAtomicUnit=on
      settings: LibrarySourceBlock=embreciprocals/Real Divide HDL Optimized/ForEach - Real Divide/MATLAB Function
  num_out : Outport  SampleTime=1e-08
  t_num_out : Outport  Port=2  SampleTime=1e-08
  wires:
  embreciprocals_c13_MATLAB_Function/2(t_num_out) -> t_num_out/1
  embreciprocals_c13_MATLAB_Function/1(num_out) -> num_out/1
  t_num/1 -> embreciprocals_c13_MATLAB_Function/2(t_num)
  num/1 -> embreciprocals_c13_MATLAB_Function/1(num)

== system gm_hdl_model_fixed_vnl/Subsystem1/Subsystem Reference/Real Divide HDL Optimized/ForEach - Real Divide_instance1/Normalize denominator ==
  u : Inport  OutDataTypeStr=fixdt(1, 17, 14)  SampleTime=1e-08
  validIn : Inport  Port=2  OutDataTypeStr=boolean  SampleTime=1e-08
  positiveRealNormalizer : Subsystem
  x : Outport  SampleTime=1e-08
  e : Outport  Port=2  SampleTime=1e-08
  isNegative : Outport  Port=3  SampleTime=1e-08
  validOut : Outport  Port=4  SampleTime=1e-08
  wires:
  validIn/1 -> positiveRealNormalizer/2(validIn)
  u/1 -> positiveRealNormalizer/1(u)
  positiveRealNormalizer/4(validOut) -> validOut/1
  positiveRealNormalizer/3(isNegative) -> isNegative/1
  positiveRealNormalizer/2(e) -> e/1
  positiveRealNormalizer/1(x) -> x/1

== system gm_hdl_model_fixed_vnl/Subsystem1/Subsystem Reference/Real Divide HDL Optimized/ForEach - Real Divide_instance1/Normalize numerator ==
  u : Inport  OutDataTypeStr=fixdt(1, 17, 14)  SampleTime=1e-08
  validIn : Inport  Port=2  OutDataTypeStr=boolean  SampleTime=1e-08
  positiveRealNormalizer : Subsystem
  positiveRealNormalizer_term3 : Terminator
  x : Outport  SampleTime=1e-08
  e : Outport  Port=2  SampleTime=1e-08
  isNegative : Outport  Port=3  SampleTime=1e-08
  wires:
  positiveRealNormalizer/4(validOut) -> positiveRealNormalizer_term3/1
  validIn/1 -> positiveRealNormalizer/2(validIn)
  u/1 -> positiveRealNormalizer/1(u)
  positiveRealNormalizer/3(isNegative) -> isNegative/1
  positiveRealNormalizer/2(e) -> e/1
  positiveRealNormalizer/1(x) -> x/1

== system gm_hdl_model_fixed_vnl/Subsystem1/Subsystem Reference/Real Divide HDL Optimized/ForEach - Real Divide_instance1/Shift and cast to output type ==
  x : Inport  OutDataTypeStr=fixdt(1, 17, 15)  SampleTime=1e-08
  shiftValue : Inport  Port=2  OutDataTypeStr=fixdt(1, 34, 0)  SampleTime=1e-08
  Abs : Abs  SampleTime=1e-08  OutDataTypeStr=int32  SaturateOnIntegerOverflow=off
  Cast to Union of Types : Subsystem
  Constant : Constant  Value=0  OutDataTypeStr=fixdt(1, 18, 10)  SampleTime=1e-08
  Data Type Conversion : DataTypeConversion  OutDataTypeStr=fixdt(1, 18, 10)  SampleTime=1e-08  RndMeth=Floor
  Delay1 : Delay  DelayLength=double(1)  InitialCondition=0  SampleTime=1e-08
  Delay3 : Delay  DelayLength=double(1)  InitialCondition=0  SampleTime=1e-08
  Switch : Switch  Threshold=double(0)  OutDataTypeStr=fixdt(1, 23, 15)  SampleTime=1e-08  SaturateOnIntegerOverflow=off  InputSameDT=off
  Variable Left Shift : Subsystem
  Variable Right Shift : Subsystem
  y : Outport  SampleTime=1e-08
  wires:
  Constant/1 -> Cast to Union of Types/1(Xref)
  Switch/1 -> Delay1/1
  Delay3/1 -> Switch/2
  Delay1/1 -> Data Type Conversion/1
  Cast to Union of Types/1(Cout) -> Variable Right Shift/1(x), Variable Left Shift/1(x)
  Abs/1 -> Variable Left Shift/2(leftShift), Variable Right Shift/2(rightShift)
  shiftValue/1 -> Delay3/1, Abs/1
  x/1 -> Cast to Union of Types/2(Cin)
  Data Type Conversion/1 -> y/1
  Variable Left Shift/1(y) -> Switch/1
  Variable Right Shift/1(y) -> Switch/3

== system gm_hdl_model_fixed_vnl/Subsystem1/Subsystem Reference/Real Divide HDL Optimized/ForEach - Real Divide_instance1/Upcast Wordlength ==
  x : Inport  OutDataTypeStr=fixdt(1, 17, 14)  SampleTime=5e-09
  y : Inport  Port=2  OutDataTypeStr=fixdt(1, 17, 14)  SampleTime=5e-09
  slutils_c2_Upcast_Wordlength : MATLAB Function
      settings: LibrarySourceBlock=slutils/Upcast Wordlength
  u : Outport  SampleTime=5e-09
  v : Outport  Port=2  SampleTime=5e-09
  wires:
  slutils_c2_Upcast_Wordlength/2(v) -> v/1
  slutils_c2_Upcast_Wordlength/1(u) -> u/1
  y/1 -> slutils_c2_Upcast_Wordlength/2(y)
  x/1 -> slutils_c2_Upcast_Wordlength/1(x)

== system gm_hdl_model_fixed_vnl/Subsystem1/myRMS/CORDIC Square Root HDL Optimized/Synchronous Subsystem/cordicSquareRootHDL ==
  u : Inport  OutDataTypeStr=fixdt(0, 16, 7)  PortDimensions=1  SampleTime=1e-08
  validIn : Inport  Port=2  OutDataTypeStr=boolean  PortDimensions=1  SampleTime=1e-08
  restart : Inport  Port=3  OutDataTypeStr=boolean  PortDimensions=1  SampleTime=1e-08
  delayMatch : Delay  DelayLength=double(2)  InitialCondition=0  SampleTime=1e-08
  delayMatch1 : Delay  DelayLength=double(2)  InitialCondition=0  SampleTime=1e-08
  embmathops_c2_s84XJG1CWMolALoedlonStG_cordicSquareRootHDL_controlled : Subsystem
  stateControl : Constant  OutDataTypeStr=boolean  SampleTime=1e-08
  dataOut : Outport  SampleTime=1e-08  VectorParamsAs1DForOutWhenUnconnected=off
  eOut : Outport  Port=2  SampleTime=1e-08
  isZero : Outport  Port=3  SampleTime=1e-08
  validOut : Outport  Port=4  SampleTime=1e-08
  wires:
  stateControl/1 -> delayMatch1/1
  restart/1 -> delayMatch/1
  delayMatch1/1 -> embmathops_c2_s84XJG1CWMolALoedlonStG_cordicSquareRootHDL_controlled/Enable
  embmathops_c2_s84XJG1CWMolALoedlonStG_cordicSquareRootHDL_controlled/4(out3) -> validOut/1
  embmathops_c2_s84XJG1CWMolALoedlonStG_cordicSquareRootHDL_controlled/3(out2) -> isZero/1
  embmathops_c2_s84XJG1CWMolALoedlonStG_cordicSquareRootHDL_controlled/2(out1) -> eOut/1
  embmathops_c2_s84XJG1CWMolALoedlonStG_cordicSquareRootHDL_controlled/1(out0) -> dataOut/1
  delayMatch/1 -> embmathops_c2_s84XJG1CWMolALoedlonStG_cordicSquareRootHDL_controlled/3(in2)
  validIn/1 -> embmathops_c2_s84XJG1CWMolALoedlonStG_cordicSquareRootHDL_controlled/2(in1)
  u/1 -> embmathops_c2_s84XJG1CWMolALoedlonStG_cordicSquareRootHDL_controlled/1(in0)

== system gm_hdl_model_fixed_vnl/Subsystem1/Subsystem Reference/Absolute of Complex/CORDIC Square Root HDL Optimized1/Synchronous Subsystem/cordicSquareRootHDL ==
  u : Inport  OutDataTypeStr=fixdt(1, 24, 22)  PortDimensions=1  SampleTime=5e-09
  validIn : Inport  Port=2  OutDataTypeStr=boolean  PortDimensions=1  SampleTime=1e-08
  restart : Inport  Port=3  OutDataTypeStr=boolean  PortDimensions=1  SampleTime=1e-08
  RateTransition : RateTransition  OutPortSampleTimeOpt=Multiple of input port sample time  OutPortSampleTimeMultiple=2
  crp_out : Delay  DelayLength=double(1)  InitialCondition=0  SampleTime=5e-09
  delayMatch : Delay  DelayLength=double(2)  InitialCondition=0  SampleTime=1e-08
  delayMatch1 : Delay  DelayLength=double(2)  InitialCondition=0  SampleTime=1e-08
  delayMatch2 : Delay  DelayLength=double(2)  InitialCondition=0  SampleTime=1e-08
  embmathops_c2_srwrzER3uCGRdPfDbow0ID_cordicSquareRootHDL_controlled : Subsystem
  stateControl : Constant  OutDataTypeStr=boolean  SampleTime=1e-08
  dataOut : Outport  SampleTime=1e-08  VectorParamsAs1DForOutWhenUnconnected=off
  eOut : Outport  Port=2  SampleTime=1e-08
  isZero : Outport  Port=3  SampleTime=1e-08
  validOut : Outport  Port=4  SampleTime=1e-08
  wires:
  stateControl/1 -> delayMatch2/1
  restart/1 -> delayMatch1/1
  validIn/1 -> delayMatch/1
  delayMatch2/1 -> embmathops_c2_srwrzER3uCGRdPfDbow0ID_cordicSquareRootHDL_controlled/Enable
  RateTransition/1 -> embmathops_c2_srwrzER3uCGRdPfDbow0ID_cordicSquareRootHDL_controlled/1(in0)
  u/1 -> crp_out/1
  crp_out/1 -> RateTransition/1
  embmathops_c2_srwrzER3uCGRdPfDbow0ID_cordicSquareRootHDL_controlled/4(out3) -> validOut/1
  embmathops_c2_srwrzER3uCGRdPfDbow0ID_cordicSquareRootHDL_controlled/3(out2) -> isZero/1
  embmathops_c2_srwrzER3uCGRdPfDbow0ID_cordicSquareRootHDL_controlled/2(out1) -> eOut/1
  embmathops_c2_srwrzER3uCGRdPfDbow0ID_cordicSquareRootHDL_controlled/1(out0) -> dataOut/1
  delayMatch1/1 -> embmathops_c2_srwrzER3uCGRdPfDbow0ID_cordicSquareRootHDL_controlled/3(in2)
  delayMatch/1 -> embmathops_c2_srwrzER3uCGRdPfDbow0ID_cordicSquareRootHDL_controlled/2(in1)

== system gm_hdl_model_fixed_vnl/Subsystem1/Subsystem Reference/CORDIC Square Root HDL Optimized/Synchronous Subsystem/cordicSquareRootHDL/embmathops_c2_skVmLPFzLIK224pVNfQB1qF_cordicSquareRootHDL_controlled ==
  in0 : Inport  OutDataTypeStr=fixdt(1, 22, 20)  SampleTime=1e-08
  in1 : Inport  Port=2  OutDataTypeStr=boolean  SampleTime=1e-08
  in2 : Inport  Port=3  OutDataTypeStr=boolean  SampleTime=1e-08
  stateControl : EnablePort  OutDataTypeStr=boolean
  embmathops_c2_skVmLPFzLIK224pVNfQB1qF_cordicSquareRootHDL : MATLAB Function  TreatAsAtomicUnit=on
      settings: LibrarySourceBlock=embmathops/CORDIC Square Root HDL Optimized/Synchronous Subsystem/cordicSquareRootHDL
  out0 : Outport  OutDataTypeStr=fixdt(1, 22, 20)  SampleTime=1e-08  InitialOutput=0
  out1 : Outport  Port=2  OutDataTypeStr=int32  SampleTime=1e-08  InitialOutput=0
  out2 : Outport  Port=3  OutDataTypeStr=boolean  SampleTime=1e-08  InitialOutput=0
  out3 : Outport  Port=4  OutDataTypeStr=boolean  SampleTime=1e-08  InitialOutput=0
  wires:
  in2/1 -> embmathops_c2_skVmLPFzLIK224pVNfQB1qF_cordicSquareRootHDL/3(restart)
  in1/1 -> embmathops_c2_skVmLPFzLIK224pVNfQB1qF_cordicSquareRootHDL/2(validIn)
  in0/1 -> embmathops_c2_skVmLPFzLIK224pVNfQB1qF_cordicSquareRootHDL/1(u)
  embmathops_c2_skVmLPFzLIK224pVNfQB1qF_cordicSquareRootHDL/4(validOut) -> out3/1
  embmathops_c2_skVmLPFzLIK224pVNfQB1qF_cordicSquareRootHDL/3(isZero) -> out2/1
  embmathops_c2_skVmLPFzLIK224pVNfQB1qF_cordicSquareRootHDL/2(eOut) -> out1/1
  embmathops_c2_skVmLPFzLIK224pVNfQB1qF_cordicSquareRootHDL/1(dataOut) -> out0/1

== system gm_hdl_model_fixed_vnl/Subsystem1/Subsystem Reference/Real Divide HDL Optimized/ForEach - Real Divide_instance1/Divide by zero handler/Compare To Zero ==
  u : Inport  OutDataTypeStr=fixdt(1, 17, 15)  SampleTime=1e-08
  Compare : RelationalOperator  OutDataTypeStr=boolean
  Constant : Constant  DisableCoverage=on  Value=0  OutDataTypeStr=fixdt(1, 17, 15)  SampleTime=-1  PreserveConstantTs=on
  y : Outport  SampleTime=1e-08
  wires:
  u/1 -> Compare/1
  Compare/1 -> y/1
  Constant/1 -> Compare/2

== system gm_hdl_model_fixed_vnl/Subsystem1/Subsystem Reference/Real Divide HDL Optimized/ForEach - Real Divide_instance1/Divide real numerator by denominator/normalizedCORDICDivide ==
  num : Inport  OutDataTypeStr=fixdt(1, 17, 15)  PortDimensions=1  SampleTime=1e-08
  den : Inport  Port=2  OutDataTypeStr=fixdt(1, 17, 15)  PortDimensions=1  SampleTime=1e-08
  tNum : Inport  Port=3  OutDataTypeStr=fixdt(1, 33, 0)  PortDimensions=1  SampleTime=1e-08
  tDen : Inport  Port=4  OutDataTypeStr=int32  PortDimensions=1  SampleTime=1e-08
  isNumNegative : Inport  Port=5  OutDataTypeStr=boolean  PortDimensions=1  SampleTime=1e-08
  isDenNegative : Inport  Port=6  OutDataTypeStr=boolean  PortDimensions=1  SampleTime=1e-08
  validIn : Inport  Port=7  OutDataTypeStr=boolean  PortDimensions=1  SampleTime=1e-08
  delayMatch : Delay  DelayLength=double(5)  InitialCondition=0  SampleTime=1e-08
  embreciprocals_c21_normalizedCORDICDivide_controlled : Subsystem
  stateControl : Constant  OutDataTypeStr=boolean  SampleTime=1e-08
  y : Outport  SampleTime=1e-08  VectorParamsAs1DForOutWhenUnconnected=off
  t : Outport  Port=2  SampleTime=1e-08  VectorParamsAs1DForOutWhenUnconnected=off
  isDenZeroOut : Outport  Port=3  SampleTime=1e-08
  validOut : Outport  Port=4  SampleTime=1e-08  VectorParamsAs1DForOutWhenUnconnected=off
  wires:
  stateControl/1 -> delayMatch/1
  delayMatch/1 -> embreciprocals_c21_normalizedCORDICDivide_controlled/Enable
  embreciprocals_c21_normalizedCORDICDivide_controlled/4(out3) -> validOut/1
  embreciprocals_c21_normalizedCORDICDivide_controlled/3(out2) -> isDenZeroOut/1
  embreciprocals_c21_normalizedCORDICDivide_controlled/2(out1) -> t/1
  embreciprocals_c21_normalizedCORDICDivide_controlled/1(out0) -> y/1
  validIn/1 -> embreciprocals_c21_normalizedCORDICDivide_controlled/7(in6)
  isDenNegative/1 -> embreciprocals_c21_normalizedCORDICDivide_controlled/6(in5)
  isNumNegative/1 -> embreciprocals_c21_normalizedCORDICDivide_controlled/5(in4)
  tDen/1 -> embreciprocals_c21_normalizedCORDICDivide_controlled/4(in3)
  tNum/1 -> embreciprocals_c21_normalizedCORDICDivide_controlled/3(in2)
  den/1 -> embreciprocals_c21_normalizedCORDICDivide_controlled/2(in1)
  num/1 -> embreciprocals_c21_normalizedCORDICDivide_controlled/1(in0)
